simulink model "Thermal_Household_Model"  (R2022a)
settings: Solver=VariableStepAuto  StartTime=0.0  StopTime=86400*7  RelTol=1e-3
settings Model: Creator=matm  LastModifiedBy=nikos
settings SolverCC: ShapePreserveControl=EnableAll  AlgebraicLoopSolver=TrustRegion  SolverResetMethod=Robust
settings DataIOCC: ReturnWorkspaceOutputs=off
settings DebuggingCC: UnconnectedInputMsg=warning  UnconnectedOutputMsg=warning  UnconnectedLineMsg=warning  SFMachineParentedDataDiag=warning  ArithmeticOperatorsInVariantConditions=warning
settings SFSimCC: SimUseLocalCustomCode=off  CustomCodeUndefinedFunction=UseInterfaceOnly
settings RTWCC: RTWUseLocalCustomCode=off
settings CodeAppCC: StateflowObjectComments=on

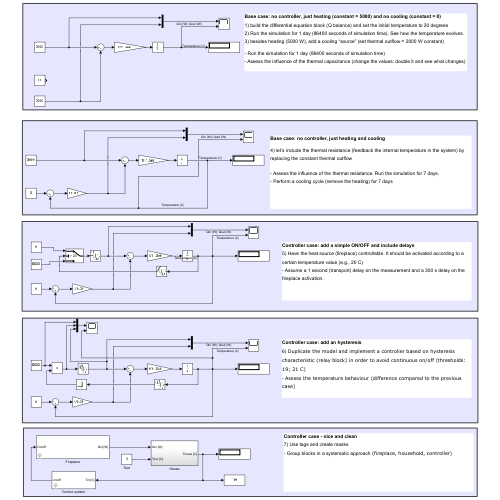
[thumbnail: Simulink's stored preview of the top-level diagram]
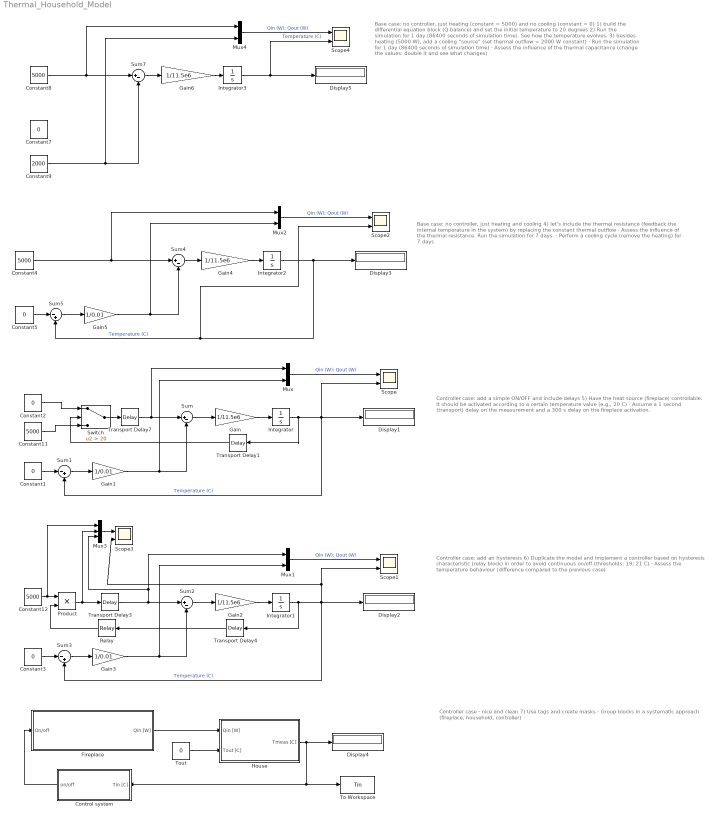
== system Thermal_Household_Model ==
  note: Controller case: add a simple ON/OFF and include delays
      | 5) Have the heat source (fireplace) controllable. It should be activated according to a certain temperature value (e.g., 20 C)
      | - Assume a 1 second (transport) delay on the measurement and a 300 s delay on the fireplace activation.
  note: Base case: no controller, just heating and cooling
      |
      | 4) let’s include the thermal resistance (feedback the internal temperature in the system) by replacing the constant thermal outflow
      |
      | - Assess the influence of the thermal resistance. Run the simulation for 7 days.
      | - Perform a cooling cycle (remove the heating) for 7 days
  note: Base case: no controller, just heating (constant = 5000) and no cooling (constant = 0)
      | 1) build the differential equation block (Q balance) and set the initial temperature to 20 degrees
      | 2) Run the simulation for 1 day (86400 seconds of simulation time). See how the temperature evolves.
      | 3) besides heating (5000 W), add a cooling “source” (set thermal outflow = 2000 W constant)
      |
      | - Run the simulation for 1 day (86400 seconds of simulation time)
      | - Assess the influence of the thermal capacitance (change the values: double it and see what changes)
  note: Controller case: add an hysteresis
      | 6) Duplicate the model and implement a controller based on hysteresis characteristic (relay block) in order to avoid continuous on/off (thresholds: 19; 21 C)
      | - Assess the temperature behaviour (difference compared to the previous case)
  note: Controller case - nice and clean
      | 7) Use tags and create masks
      | - Group blocks in a systematic approach (fireplace, household, controller)
  Constant{1..3,5,7} (5 alike) : Constant  Value=0
  Constant{4,8,11..12} (4 alike) : Constant  Value=5000
  Constant9 : Constant  Value=2000
  Control system : Subsystem  mask{Ton=19, Toff=21, Tmeas=1}
      mask prompts: Ton "Switch on temperature [C]"; Toff "Switch off temperature [C]"; Tmeas "Measurement time [s]"
      mask DialogControl DescGroupVar Prompt: Control and measurement system
  Display{1..5} (5 alike) : Display
  Fireplace : Subsystem  mask{Pfire=5000, Tstart=300}
      mask prompts: Pfire "Fireplace power [W]"; Tstart "Starting time [s]"
      mask DialogControl DescGroupVar Prompt: Fireplace
      mask DialogControl DescTextVar Prompt: A 5 kW fireplace is modelled
  Gain{,2,4,6} (4 alike) : Gain  Gain=1/11.5e6
  Gain1 : Gain  Gain=1/0.01
  Gain3 : Gain  Gain=1/0.01
  Gain5 : Gain  Gain=1/0.01
  House : Subsystem
  Integrator : Integrator  InitialCondition=18
  Integrator1 : Integrator  InitialCondition=18
  Integrator2 : Integrator  InitialCondition=20
  Integrator3 : Integrator  InitialCondition=20
  Mux{,1..2,4} (4 alike) : Mux  Inputs=2
  Mux3 : Mux  Inputs=3
  Product : Product
  Relay : Relay  OnSwitchValue=21  OffSwitchValue=19  OnOutputValue=0  OffOutputValue=1  ZeroCross=off
  Scope{,1..4} (5 alike) : Scope  NumInputPorts=2
  Sum{,2,4,7} (4 alike) : Sum  Inputs=|+-
  Sum1 : Sum  Inputs=|-+
  Sum3 : Sum  Inputs=|-+
  Sum5 : Sum  Inputs=|-+
  Switch : Switch  Criteria=u2 > Threshold  Threshold=20  ZeroCross=off  SaturateOnIntegerOverflow=off  InputSameDT=off
  To Workspace : ToWorkspace  VariableName=Tin  SaveFormat=Structure With Time  SampleTime=1
  Tout : Constant  Value=0
  Transport Delay1 : TransportDelay  InitialOutput=18
  Transport Delay3 : TransportDelay  DelayTime=300
  Transport Delay4 : TransportDelay
  Transport Delay7 : TransportDelay  DelayTime=300
  wires:
  Integrator/1 -> Transport Delay1/1, Sum1/2, Display1/1, Scope/2  "Temperature (C)"
  Sum/1 -> Gain/1
  Gain/1 -> Integrator/1
  Mux/1 -> Scope/1  "Qin (W); Qout (W)"
  Constant1/1 -> Sum1/1
  Sum1/1 -> Gain1/1
  Gain1/1 -> Mux/2, Sum/2
  Constant11/1 -> Switch/3
  Constant2/1 -> Switch/1
  Integrator2/1 -> Scope2/2, Sum5/2, Display3/1  "Temperature (C)"
  Sum4/1 -> Gain4/1
  Gain4/1 -> Integrator2/1
  Mux2/1 -> Scope2/1  "Qin (W); Qout (W)"
  Constant5/1 -> Sum5/1
  Sum5/1 -> Gain5/1
  Gain5/1 -> Sum4/2, Mux2/2
  Integrator1/1 -> Transport Delay4/1, Scope3/2, Scope1/2, Display2/1, Sum3/2  "Temperature (C)"
  Sum2/1 -> Gain2/1
  Gain2/1 -> Integrator1/1
  Mux1/1 -> Scope1/1  "Qin (W); Qout (W)"
  Constant3/1 -> Sum3/1
  Sum3/1 -> Gain3/1
  Gain3/1 -> Sum2/2, Mux1/2
  Constant12/1 -> Mux3/1, Product/1
  Product/1 -> Mux3/2, Transport Delay3/1
  Transport Delay3/1 -> Sum2/1, Mux3/3, Mux1/1
  Relay/1 -> Product/2
  Mux3/1 -> Scope3/1
  Control system/1(on/off) -> Fireplace/1(On/off)
  Fireplace/1(Qin [W]) -> House/1(Qin [W])
  Tout/1 -> House/2(Tout [C])
  House/1(Tmeas [C]) -> To Workspace/1, Control system/1(Tin [C]), Display4/1
  Integrator3/1 -> Scope4/2, Display5/1  "Temperature (C)"
  Sum7/1 -> Gain6/1
  Gain6/1 -> Integrator3/1
  Mux4/1 -> Scope4/1  "Qin (W); Qout (W)"
  Constant8/1 -> Sum7/1, Mux4/1
  Switch/1 -> Transport Delay7/1
  Constant4/1 -> Mux2/1, Sum4/1
  Transport Delay7/1 -> Mux/1, Sum/1
  Transport Delay4/1 -> Relay/1
  Transport Delay1/1 -> Switch/2
  Constant9/1 -> Mux4/2, Sum7/2

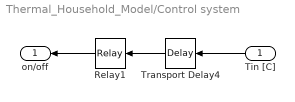
== system Thermal_Household_Model/Control system ==
  Tin [C] : Inport
  Relay1 : Relay  OnSwitchValue=Toff  OffSwitchValue=Ton  OnOutputValue=0  OffOutputValue=1  ZeroCross=off
  Transport Delay4 : TransportDelay  DelayTime=Tmeas
  on/off : Outport  VectorParamsAs1DForOutWhenUnconnected=off
  wires:
  Tin [C]/1 -> Transport Delay4/1
  Relay1/1 -> on/off/1
  Transport Delay4/1 -> Relay1/1

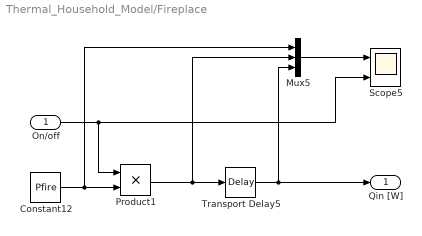
== system Thermal_Household_Model/Fireplace ==
  On/off : Inport
  Constant12 : Constant  Value=Pfire
  Mux5 : Mux  Inputs=3
  Product1 : Product
  Scope5 : Scope  NumInputPorts=2
  Transport Delay5 : TransportDelay  DelayTime=Tstart
  Qin [W] : Outport  VectorParamsAs1DForOutWhenUnconnected=off
  wires:
  Constant12/1 -> Product1/2, Mux5/1
  Product1/1 -> Transport Delay5/1, Mux5/2
  Transport Delay5/1 -> Mux5/3, Qin [W]/1
  Mux5/1 -> Scope5/1
  On/off/1 -> Scope5/2, Product1/1

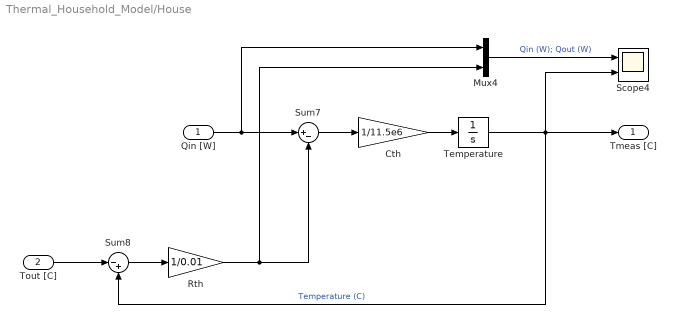
== system Thermal_Household_Model/House ==
  Qin [W] : Inport
  Tout [C] : Inport  Port=2
  Cth : Gain  Gain=1/11.5e6
  Mux4 : Mux  Inputs=2
  Rth : Gain  Gain=1/0.01
  Scope4 : Scope  NumInputPorts=2
  Sum7 : Sum  Inputs=|+-
  Sum8 : Sum  Inputs=|-+
  Temperature : Integrator  InitialCondition=18
  Tmeas [C] : Outport  VectorParamsAs1DForOutWhenUnconnected=off
  wires:
  Temperature/1 -> Sum8/2, Tmeas [C]/1, Scope4/2  "Temperature (C)"
  Sum7/1 -> Cth/1
  Cth/1 -> Temperature/1
  Mux4/1 -> Scope4/1  "Qin (W); Qout (W)"
  Tout [C]/1 -> Sum8/1
  Sum8/1 -> Rth/1
  Rth/1 -> Mux4/2, Sum7/2
  Qin [W]/1 -> Mux4/1, Sum7/1
